simulink model "sampleModel1488"  (R2023a)
settings: Solver=VariableStepAuto  StartTime=0.0  StopTime=10.0  RelTol=1e-3
undefined symbols (not defined in the file): b011101a, b0c8, bf87616c, DiscIntNeverNeededParam, Newton, Raphson
libraries: simulink x171, slpidlib x32, simulink_need_slupdate x2
(part 2 of 6)

== system sampleModel1488/cfblk140 ==
  cfblk1 : Inport
  cfblk9 : Inport  Port=2
  cfblk10 : Inport  Port=3
  cfblk11 : Inport  Port=4
  cfblk14 : Delay  SampleTime=1
  cfblk3 : simulink/Discrete/Tapped Delay  vinit=0.0  samptime=-1  NumDelays=1  DelayOrder=Oldest  includeCurrent=off
  cfblk4 : Delay  SampleTime=1
  cfblk5 : Assignment  DiagnosticForDimensions=Warning  IndexOptions=Index vector (dialog)  Indices=1  OutputSizes=1
  cfblk6 : Gain  Gain=[-337675472.519738]
  cfblk7 : Subsystem
  cfblk8 : Subsystem
  cfblk2 : Outport
  cfblk12 : Outport  Port=2
  cfblk13 : Outport  Port=3
  wires:
  cfblk1/1 -> cfblk12/1
  cfblk8/1(cfblk2) -> cfblk2/1
  cfblk4/1 -> cfblk6/1
  cfblk9/1 -> cfblk4/1
  cfblk10/1 -> cfblk7/1(cfblk1)
  cfblk3/1 -> cfblk8/1(cfblk1)
  cfblk11/1 -> cfblk5/1
  cfblk8/2(cfblk11) -> cfblk5/2
  cfblk6/1 -> cfblk7/2(cfblk11), cfblk7/3(cfblk12)
  cfblk7/1(cfblk2) -> cfblk8/2(cfblk10)
  cfblk7/2(cfblk13) -> cfblk13/1
  cfblk5/1 -> cfblk14/1
  cfblk14/1 -> cfblk3/1

== system sampleModel1488/cfblk141 ==
  cfblk1 : Inport
  cfblk12 : Inport  Port=2
  cfblk13 : Inport  Port=3
  cfblk10 : Subsystem
  cfblk11 : Subsystem
  cfblk14 : Delay  SampleTime=1
  cfblk15 : Delay  SampleTime=1
  cfblk3 : Delay  SampleTime=1
  cfblk4 : PermuteDimensions
  cfblk5 : Signum
  cfblk6 : Math
  cfblk7 : Constant  Value=[773437629.546619]  SampleTime=1
  cfblk8 : Constant  Value=[-615309156.626634]  SampleTime=1
  cfblk9 : Subsystem
  cfblk2 : Outport
  wires:
  cfblk12/1 -> cfblk4/1
  cfblk11/2(cfblk7) -> cfblk10/1(cfblk1)
  cfblk8/1 -> cfblk2/1
  cfblk7/1 -> cfblk5/1
  cfblk1/1 -> cfblk9/2(cfblk7)
  cfblk13/1 -> cfblk9/3(cfblk8)
  cfblk9/1(cfblk2) -> cfblk3/1
  cfblk9/2(cfblk10) -> cfblk6/1
  cfblk4/1 -> cfblk11/1(cfblk1)
  cfblk9/3(cfblk11) -> cfblk11/2(cfblk6)
  cfblk11/1(cfblk2) -> cfblk14/1
  cfblk14/1 -> cfblk9/1(cfblk1)
  cfblk10/1(cfblk2) -> cfblk15/1
  cfblk15/1 -> cfblk9/4(cfblk9)

== system sampleModel1488/cfblk142 ==
  cfblk1 : Inport
  cfblk8 : Inport  Port=2
  cfblk{10..14} (5 alike) : Delay  SampleTime=1
  cfblk3 : Constant  Value=[-728485137.526243]  SampleTime=1
  cfblk4 : Subsystem
  cfblk5 : Subsystem
  cfblk6 : Subsystem
  cfblk7 : Subsystem
  cfblk2 : Outport
  cfblk9 : Outport  Port=2
  wires:
  cfblk8/1 -> cfblk2/1, cfblk6/3(cfblk13), cfblk6/6(cfblk16)
  cfblk5/1(cfblk2) -> cfblk7/1(cfblk1)
  cfblk1/1 -> cfblk4/1(cfblk1), cfblk6/2(cfblk12)
  cfblk5/2(cfblk8) -> cfblk13/1, cfblk14/1
  cfblk3/1 -> cfblk4/3(cfblk14)
  cfblk4/1(cfblk2) -> cfblk9/1
  cfblk6/1(cfblk2) -> cfblk5/2(cfblk6)
  cfblk4/2(cfblk15) -> cfblk6/1(cfblk1)
  cfblk7/2(cfblk15) -> cfblk11/1, cfblk12/1
  cfblk7/1(cfblk2) -> cfblk10/1
  cfblk10/1 -> cfblk5/1(cfblk1)
  cfblk11/1 -> cfblk5/3(cfblk7)
  cfblk12/1 -> cfblk6/5(cfblk15)
  cfblk13/1 -> cfblk4/2(cfblk13)
  cfblk14/1 -> cfblk6/4(cfblk14)

== system sampleModel1488/cfblk143 ==
  cfblk1 : Inport
  cfblk11 : Inport  Port=2
  cfblk10 : Subsystem
  cfblk12 : Delay  SampleTime=1
  cfblk13 : Delay  SampleTime=1
  cfblk3 : simulink/Discrete/Transfer Fcn First Order  PoleZ=0.95  ICPrevOutput=0.0  DoSatur=off
  cfblk4 : DiscreteFir  SampleTime=1
  cfblk5 : Squeeze
  cfblk6 : ComplexToRealImag
  cfblk7 : Subsystem
  cfblk8 : Subsystem
  cfblk9 : Subsystem
  cfblk2 : Outport
  wires:
  cfblk1/1 -> cfblk9/1(cfblk1)
  cfblk8/1(cfblk2) -> cfblk6/1
  cfblk8/2(cfblk8) -> cfblk2/1
  cfblk4/1 -> cfblk10/1(cfblk1)
  cfblk9/1(cfblk2) -> cfblk4/1
  cfblk7/1(cfblk2) -> cfblk5/1
  cfblk10/1(cfblk2) -> cfblk3/1
  cfblk5/1 -> cfblk8/1(cfblk1)
  cfblk7/2(cfblk13) -> cfblk8/2(cfblk7)
  cfblk11/1 -> cfblk7/1(cfblk1)
  cfblk9/2(cfblk12) -> cfblk7/2(cfblk9)
  cfblk3/1 -> cfblk7/3(cfblk10)
  cfblk10/2(cfblk8) -> cfblk7/5(cfblk12)
  cfblk6/1 -> cfblk12/1
  cfblk12/1 -> cfblk10/2(cfblk7)
  cfblk6/2 -> cfblk13/1
  cfblk13/1 -> cfblk7/4(cfblk11)

== system sampleModel1488/cfblk144 ==
  cfblk1 : Inport
  cfblk3 : DiscreteZeroPole  Poles=[0 0.5]  Gain=1
  cfblk4 : DiscreteZeroPole  Poles=[0 0.5]  Gain=1
  cfblk5 : Polyval  Coefs=[ +2.081618890e-019, -1.441693666e-014, +4.719686976e-010, -8.536869453e-006, +1.621573104e-001, -8.087801117e+001 ]
  cfblk6 : Signum
  cfblk7 : Product  Inputs=**
  cfblk9 : Delay  SampleTime=1
  cfblk2 : Outport
  cfblk8 : Outport  Port=2
  wires:
  cfblk5/1 -> cfblk2/1
  cfblk4/1 -> cfblk6/1
  cfblk7/1 -> cfblk4/1
  cfblk3/1 -> cfblk8/1, cfblk9/1
  cfblk6/1 -> cfblk3/1, cfblk5/1
  cfblk1/1 -> cfblk7/2
  cfblk9/1 -> cfblk7/1

== system sampleModel1488/cfblk145 ==
  cfblk1 : Inport
  cfblk9 : Inport  Port=2
  cfblk10 : Inport  Port=3
  cfblk11 : Inport  Port=4
  cfblk12 : Delay  SampleTime=1
  cfblk13 : Delay  SampleTime=1
  cfblk3 : Delay  DelayLengthSource=Input port  SampleTime=1
      settings: InputPortMap=u0,p1
  cfblk4 : DiscreteFilter  SampleTime=1
  cfblk5 : Bias  Bias=[63106106.274420]  SaturateOnIntegerOverflow=off
  cfblk6 : Constant  Value=[428304277.338585]  SampleTime=1
  cfblk7 : Subsystem
  cfblk8 : Subsystem
  cfblk2 : Outport
  wires:
  cfblk11/1 -> cfblk3/1
  cfblk6/1 -> cfblk7/1(cfblk1)
  cfblk5/1 -> cfblk7/2(cfblk11)
  cfblk9/1 -> cfblk2/1
  cfblk4/1 -> cfblk8/1(cfblk1)
  cfblk10/1 -> cfblk8/2(cfblk9)
  cfblk8/1(cfblk2) -> cfblk5/1
  cfblk1/1 -> cfblk3/2
  cfblk7/1(cfblk2) -> cfblk12/1
  cfblk12/1 -> cfblk4/1
  cfblk7/2(cfblk12) -> cfblk13/1
  cfblk13/1 -> cfblk8/3(cfblk10)

== system sampleModel1488/cfblk146 ==
  cfblk1 : Inport
  cfblk10 : Subsystem
  cfblk11 : Delay  SampleTime=1
  cfblk12 : Delay  SampleTime=1
  cfblk13 : Delay  SampleTime=1
  cfblk3 : simulink/Discrete/Transfer Fcn Real Zero  ZeroZ=0.75  ICPrevInput=0.0  DoSatur=off
  cfblk4 : Sqrt  Operator=rSqrt  AlgorithmType=Newton-Raphson
  cfblk5 : Constant  Value=[-692942058.607273]  SampleTime=1
  cfblk6 : Subsystem
  cfblk7 : Subsystem
  cfblk8 : Subsystem
  cfblk9 : Subsystem
  cfblk2 : Outport
  wires:
  cfblk10/1(cfblk2) -> cfblk6/2(cfblk12)
  cfblk8/1(cfblk2) -> cfblk3/1
  cfblk8/2(cfblk10) -> cfblk9/1(cfblk1)
  cfblk1/1 -> cfblk7/2(cfblk9)
  cfblk6/1(cfblk2) -> cfblk4/1
  cfblk7/1(cfblk2) -> cfblk2/1
  cfblk7/2(cfblk10) -> cfblk8/1(cfblk1)
  cfblk9/3(cfblk15) -> cfblk10/1(cfblk1)
  cfblk3/1 -> cfblk10/2(cfblk9)
  cfblk4/1 -> cfblk11/1
  cfblk11/1 -> cfblk6/1(cfblk1)
  cfblk9/1(cfblk2) -> cfblk12/1
  cfblk12/1 -> cfblk7/1(cfblk1)
  cfblk9/2(cfblk14) -> cfblk13/1
  cfblk13/1 -> cfblk8/2(cfblk9)

== system sampleModel1488/cfblk147 ==
  cfblk1 : Inport
  cfblk10 : Subsystem
  cfblk11 : Subsystem
  cfblk{12..15} (4 alike) : Delay  SampleTime=1
  cfblk3 : Delay  ShowEnablePort=on  SampleTime=1
      settings: InputPortMap=u0,e6
  cfblk4 : UnitDelay  HasFrameUpgradeWarning=on
  cfblk5 : Sum  Inputs=+
  cfblk6 : Assignment  DiagnosticForDimensions=Warning  IndexOptions=Index vector (dialog)  Indices=1  OutputSizes=1
  cfblk7 : PermuteDimensions
  cfblk8 : Constant  Value=[-634312519.623233]  SampleTime=1
  cfblk9 : Subsystem
  cfblk2 : Outport
  wires:
  cfblk3/1 -> cfblk5/1
  cfblk4/1 -> cfblk10/1(cfblk1), cfblk9/3(cfblk8)
  cfblk11/1(cfblk2) -> cfblk3/1
  cfblk11/2(cfblk8) -> cfblk7/1
  cfblk1/1 -> cfblk2/1, cfblk11/3(cfblk6), cfblk11/4(cfblk7)
  cfblk9/1(cfblk2) -> cfblk13/1, cfblk14/1
  cfblk10/1(cfblk2) -> cfblk9/5(cfblk10), cfblk12/1
  cfblk7/1 -> cfblk4/1
  cfblk5/1 -> cfblk10/3(cfblk9)
  cfblk8/1 -> cfblk6/1, cfblk9/1(cfblk1), cfblk9/2(cfblk7), cfblk10/4(cfblk10)
  cfblk11/3(cfblk9) -> cfblk6/2, cfblk9/4(cfblk9)
  cfblk12/1 -> cfblk3/2
  cfblk13/1 -> cfblk10/2(cfblk8)
  cfblk14/1 -> cfblk11/2(cfblk5)
  cfblk6/1 -> cfblk15/1
  cfblk15/1 -> cfblk11/1(cfblk1)

== system sampleModel1488/cfblk148 ==
  cfblk1 : Inport
  cfblk{10..17} (8 alike) : Delay  SampleTime=1
  cfblk3 : simulink/Math Operations/MinMax Running Resettable  Function=min  vinit=0.0
  cfblk4 : PermuteDimensions
  cfblk5 : Polyval  Coefs=[ +2.081618890e-019, -1.441693666e-014, +4.719686976e-010, -8.536869453e-006, +1.621573104e-001, -8.087801117e+001 ]
  cfblk6 : ComplexToRealImag
  cfblk7 : Subsystem
  cfblk8 : Subsystem
  cfblk2 : Outport
  cfblk9 : Outport  Port=2
  wires:
  cfblk7/1(cfblk2) -> cfblk8/1(cfblk1)
  cfblk1/1 -> cfblk7/1(cfblk1)
  cfblk3/1 -> cfblk4/1, cfblk14/1
  cfblk5/1 -> cfblk3/1, cfblk15/1
  cfblk8/1(cfblk2) -> cfblk2/1
  cfblk7/2(cfblk14) -> cfblk6/1
  cfblk4/1 -> cfblk10/1, cfblk11/1, cfblk12/1, cfblk13/1
  cfblk6/1 -> cfblk9/1
  cfblk8/2(cfblk13) -> cfblk5/1, cfblk16/1
  cfblk10/1 -> cfblk8/2(cfblk10)
  cfblk11/1 -> cfblk3/2
  cfblk12/1 -> cfblk8/3(cfblk11)
  cfblk13/1 -> cfblk7/4(cfblk12)
  cfblk14/1 -> cfblk8/4(cfblk12)
  cfblk15/1 -> cfblk7/3(cfblk11)
  cfblk16/1 -> cfblk7/5(cfblk13)
  cfblk6/2 -> cfblk17/1
  cfblk17/1 -> cfblk7/2(cfblk10)

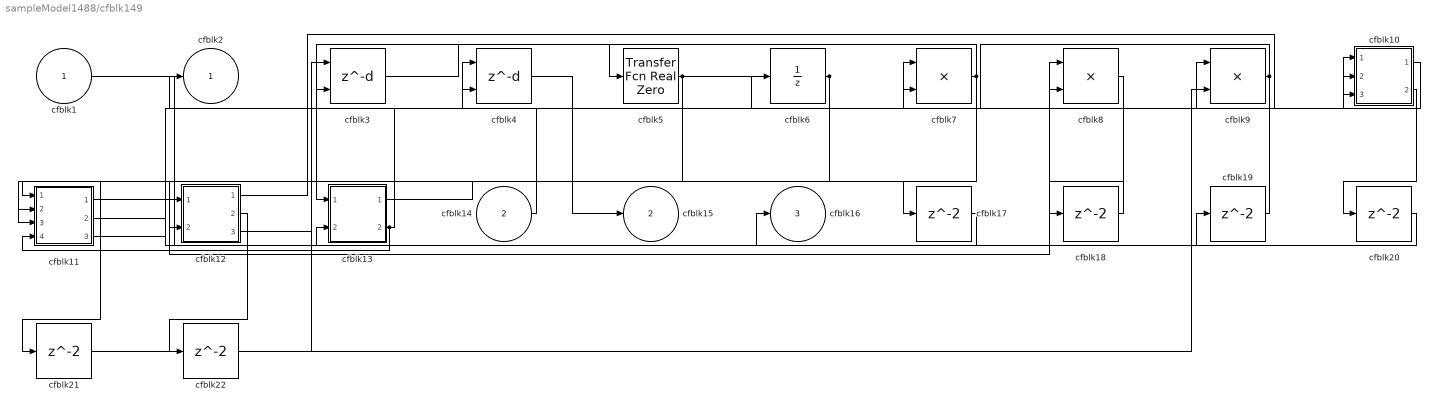
== system sampleModel1488/cfblk149 ==
  cfblk1 : Inport
  cfblk14 : Inport  Port=2
  cfblk10 : Subsystem
  cfblk11 : Subsystem
  cfblk12 : Subsystem
  cfblk13 : Subsystem
  cfblk{17..22} (6 alike) : Delay  SampleTime=1
  cfblk3 : Delay  DelayLengthSource=Input port  SampleTime=1
      settings: InputPortMap=u0,p1
  cfblk4 : Delay  DelayLengthSource=Input port  SampleTime=1
      settings: InputPortMap=u0,p1
  cfblk5 : simulink/Discrete/Transfer Fcn Real Zero  ZeroZ=0.75  ICPrevInput=0.0  DoSatur=off
  cfblk6 : UnitDelay  HasFrameUpgradeWarning=on
  cfblk7 : Product
  cfblk8 : Product
  cfblk9 : Product  Inputs=**
  cfblk2 : Outport
  cfblk15 : Outport  Port=2
  cfblk16 : Outport  Port=3
  wires:
  cfblk14/1 -> cfblk4/1
  cfblk7/1 -> cfblk13/1(cfblk1), cfblk11/3(cfblk14), cfblk21/1
  cfblk1/1 -> cfblk16/1
  cfblk11/1(cfblk2) -> cfblk8/1
  cfblk9/1 -> cfblk7/1, cfblk8/2
  cfblk4/1 -> cfblk15/1
  cfblk12/1(cfblk2) -> cfblk9/1
  cfblk6/1 -> cfblk12/1(cfblk1), cfblk11/1(cfblk1)
  cfblk12/3(cfblk10) -> cfblk10/1(cfblk1)
  cfblk10/1(cfblk2) -> cfblk4/2
  cfblk5/1 -> cfblk6/1, cfblk11/2(cfblk13), cfblk10/3(cfblk10)
  cfblk3/1 -> cfblk5/1
  cfblk11/3(cfblk17) -> cfblk10/2(cfblk9)
  cfblk13/2(cfblk15) -> cfblk2/1, cfblk11/4(cfblk15)
  cfblk13/1(cfblk2) -> cfblk17/1
  cfblk17/1 -> cfblk12/2(cfblk8)
  cfblk8/1 -> cfblk18/1
  cfblk18/1 -> cfblk7/2
  cfblk11/2(cfblk16) -> cfblk19/1
  cfblk19/1 -> cfblk3/2
  cfblk10/2(cfblk11) -> cfblk20/1
  cfblk20/1 -> cfblk13/2(cfblk14)
  cfblk21/1 -> cfblk9/2
  cfblk12/2(cfblk9) -> cfblk22/1
  cfblk22/1 -> cfblk3/1

== system sampleModel1488/cfblk150 ==
  cfblk1 : Inport
  cfblk10 : Inport  Port=2
  cfblk11 : Inport  Port=3
  cfblk12 : Inport  Port=4
  cfblk14 : Delay  SampleTime=1
  cfblk15 : Delay  SampleTime=1
  cfblk16 : Delay  SampleTime=1
  cfblk3 : Delay  DelayLengthSource=Input port  SampleTime=1
      settings: InputPortMap=u0,p1
  cfblk4 : Delay  ShowEnablePort=on  SampleTime=1
      settings: InputPortMap=u0,e6
  cfblk5 : Delay  ShowEnablePort=on  SampleTime=1
      settings: InputPortMap=u0,e6
  cfblk6 : Product
  cfblk7 : Sum  Inputs=--
  cfblk8 : Subsystem
  cfblk9 : Subsystem
  cfblk2 : Outport
  cfblk13 : Outport  Port=2
  wires:
  cfblk9/1(cfblk2) -> cfblk3/1
  cfblk8/1(cfblk2) -> cfblk9/1(cfblk1)
  cfblk3/1 -> cfblk5/1, cfblk4/2, cfblk15/1
  cfblk9/2(cfblk15) -> cfblk6/1
  cfblk12/1 -> cfblk13/1, cfblk8/4(cfblk15), cfblk8/5(cfblk16)
  cfblk11/1 -> cfblk5/2
  cfblk4/1 -> cfblk7/1
  cfblk7/1 -> cfblk2/1
  cfblk1/1 -> cfblk8/2(cfblk13), cfblk7/2, cfblk6/2
  cfblk9/3(cfblk16) -> cfblk3/2
  cfblk10/1 -> cfblk4/1
  cfblk5/1 -> cfblk14/1
  cfblk14/1 -> cfblk8/1(cfblk1)
  cfblk15/1 -> cfblk8/3(cfblk14)
  cfblk6/1 -> cfblk16/1
  cfblk16/1 -> cfblk9/2(cfblk14)

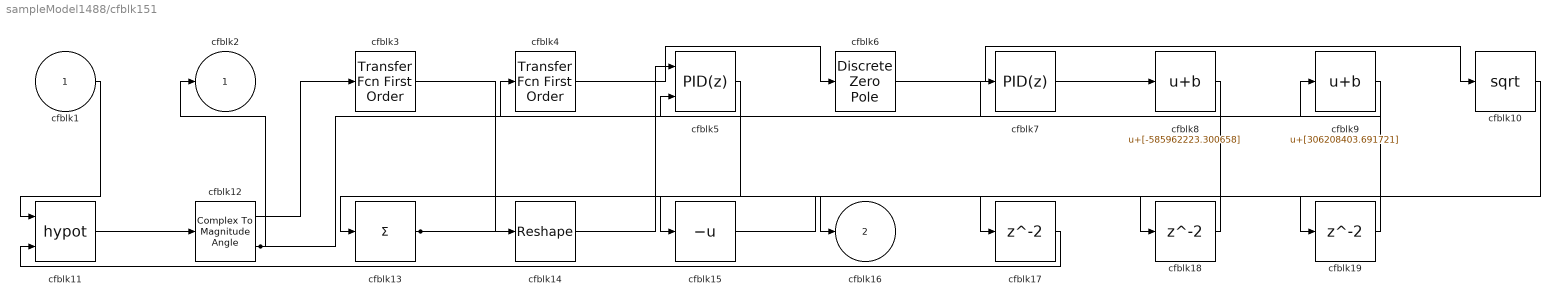
== system sampleModel1488/cfblk151 ==
  cfblk1 : Inport
  cfblk10 : Sqrt
  cfblk11 : Math  Operator=hypot
  cfblk12 : ComplexToMagnitudeAngle
  cfblk13 : Sum  Inputs=+
  cfblk14 : Reshape
  cfblk15 : UnaryMinus
  cfblk17 : Delay  SampleTime=1
  cfblk18 : Delay  SampleTime=1
  cfblk19 : Delay  SampleTime=1
  cfblk3 : simulink/Discrete/Transfer Fcn First Order  PoleZ=0.95  ICPrevOutput=0.0  DoSatur=off
  cfblk4 : simulink/Discrete/Transfer Fcn First Order  PoleZ=0.95  ICPrevOutput=0.0  DoSatur=off
  cfblk5 : slpidlib/PID Controller (2DOF)  Controller=PID  Form=Parallel  TimeDomain=Discrete-time  UseExternalTs=off  SampleTime=1  IntegratorMethod=Forward Euler  FilterMethod=Forward Euler  ControllerParametersSource=internal  P=1  I=1  UseKiTs=off  D=0  N=100  UseFilter=on  b=1  c=1  TunerSelectOption=Transfer Function Based (PID Tuner App)  InitialConditionSource=internal  InitialConditionForIntegrator=0  InitialConditionForFilter=0  DifferentiatorICPrevScaledInput=0  ExternalReset=none  TrackingMode=off  Kt=1  LimitOutput=off  SatLimitsSource=internal  UpperSaturationLimit=inf  LowerSaturationLimit=-inf  LinearizeAsGain=off  AntiWindupMode=none  Kb=1  LimitIntegrator=off  UpperIntegratorSaturationLimit=inf  LowerIntegratorSaturationLimit=-inf  POutMin=[]  POutMax=[]  IOutMin=[]  IOutMax=[]  DOutMin=[]  DOutMax=[]  NOutMin=[]  NOutMax=[]  bOutMin=[]  bOutMax=[]  cOutMin=[]  cOutMax=[]  SumOutMin=[]  SumOutMax=[]  SaturationOutMin=[]  SaturationOutMax=[]  PParamMin=[]  PParamMax=[]  IParamMin=[]  IParamMax=[]  DParamMin=[]  DParamMax=[]  NParamMin=[]  NParamMax=[]  bParamMin=[]  bParamMax=[]  cParamMin=[]  cParamMax=[]  KbParamMin=[]  KbParamMax=[]  KtParamMin=[]  KtParamMax=[]  KbOutMin=[]  KbOutMax=[]  KtOutMin=[]  KtOutMax=[]  IntegratorOutMin=[]  IntegratorOutMax=[]  FilterOutMin=[]  FilterOutMax=[]  SumI1OutMin=[]  SumI1OutMax=[]  SumI2OutMin=[]  SumI2OutMax=[]  SumI3OutMin=[]  SumI3OutMax=[]  SumI4OutMin=[]  SumI4OutMax=[]  SumDOutMin=[]  SumDOutMax=[]  Sum1OutMin=[]  Sum1OutMax=[]  Sum2OutMin=[]  Sum2OutMax=[]  Sum3OutMin=[]  Sum3OutMax=[]  DifferentiatorOutMin=[]  DifferentiatorOutMax=[]  FilterDiffOutCoefMin=[]  FilterDiffOutCoefMax=[]  ReciprocalOutMin=[]  ReciprocalOutMax=[]  SumDenOutMin=[]  SumDenOutMax=[]  SumNumOutMin=[]  SumNumOutMax=[]  DivideOutMin=[]  DivideOutMax=[]  UdiffTsProdOutMin=[]  UdiffTsProdOutMax=[]  NTsProdOutMin=[]  NTsProdOutMax=[]  UintegralTsProdOutMin=[]  UintegralTsProdOutMax=[]  UngainTsProdOutMin=[]  UngainTsProdOutMax=[]  ClampingZeroOutDataTypeStr=Inherit: Inherit via back propagation  ClampingZeroOutMin=[]  ClampingZeroOutMax=[]  FilterDenConstantOutDataTypeStr=Inherit: Inherit via back propagation  FilterDenConstantOutMin=[]  FilterDenConstantOutMax=[]  PCopyOutDataTypeStr=Inherit: Inherit via back propagation  PCopyOutMin=[]  PCopyOutMax=[]  NCopyOutDataTypeStr=Inherit: Inherit via back propagation  NCopyOutMin=[]  NCopyOutMax=[]  IntegratorContinuousStateAttributes=''  IntegratorStateMustResolveToSignalObject=off  IntegratorRTWStateStorageClass=Auto  FilterContinuousStateAttributes=''  FilterStateMustResolveToSignalObject=off  FilterRTWStateStorageClass=Auto  ParallelPVariant=InternalParameters  IdealPVariant=Disabled  IVariant=InternalParameters  DVariant=InternalParameters  bVariant=InternalParameters  cVariant=InternalParameters  IntegratorVariant=Discrete  SatVariant=Disabled  AWVariant=Passthrough  PCopyVariant=Disabled  TRVariant=Disabled  FdbkBlocksVariant=Forward  IdealPFdbkVariant=Disabled  SatFdbkVariant=Disabled  DerivativeFilterVariant=ForwardEulerFilter  NVariant=InternalParameters  NCopyVariant=Disabled  FilterICVariant=InternalICsFilter  IntegratorICVariant=InternalICs  ExternalResetVariant=Disabled  TRSumVariant=Passthrough  SumFdbkVariant=Disabled  SumVariant=Sum_PID  TsampFilterVariant=InternalTs  TsampNgainVariant=Passthrough  TsampIntegralVariant=Disabled_SignalSpec  ExternalSaturationOutDataTypeStr=Inherit: Same as second input
      settings: LibrarySourceBlock=simulink/Discrete/Discrete PID Controller (2DOF)
  cfblk6 : DiscreteZeroPole  Poles=[0 0.5]  Gain=1
  cfblk7 : slpidlib/PID Controller  Controller=PID  Form=Parallel  TimeDomain=Discrete-time  UseExternalTs=off  SampleTime=1  IntegratorMethod=Forward Euler  FilterMethod=Forward Euler  ControllerParametersSource=internal  P=1  I=1  UseKiTs=off  D=0  N=100  UseFilter=on  TunerSelectOption=Transfer Function Based (PID Tuner App)  InitialConditionSource=internal  InitialConditionForIntegrator=0  InitialConditionForFilter=0  DifferentiatorICPrevScaledInput=0  ExternalReset=none  TrackingMode=off  Kt=1  LimitOutput=off  SatLimitsSource=internal  UpperSaturationLimit=inf  LowerSaturationLimit=-inf  LinearizeAsGain=off  AntiWindupMode=none  Kb=1  LimitIntegrator=off  UpperIntegratorSaturationLimit=inf  LowerIntegratorSaturationLimit=-inf  POutMin=[]  POutMax=[]  IOutMin=[]  IOutMax=[]  DOutMin=[]  DOutMax=[]  NOutMin=[]  NOutMax=[]  SumOutMin=[]  SumOutMax=[]  SaturationOutMin=[]  SaturationOutMax=[]  PParamMin=[]  PParamMax=[]  IParamMin=[]  IParamMax=[]  DParamMin=[]  DParamMax=[]  NParamMin=[]  NParamMax=[]  KbParamMin=[]  KbParamMax=[]  KtParamMin=[]  KtParamMax=[]  KbOutMin=[]  KbOutMax=[]  KtOutMin=[]  KtOutMax=[]  IntegratorOutMin=[]  IntegratorOutMax=[]  FilterOutMin=[]  FilterOutMax=[]  SumI1OutMin=[]  SumI1OutMax=[]  SumI2OutMin=[]  SumI2OutMax=[]  SumI3OutMin=[]  SumI3OutMax=[]  SumI4OutMin=[]  SumI4OutMax=[]  SumDOutMin=[]  SumDOutMax=[]  DifferentiatorOutMin=[]  DifferentiatorOutMax=[]  FilterDiffOutCoefMin=[]  FilterDiffOutCoefMax=[]  ReciprocalOutMin=[]  ReciprocalOutMax=[]  SumDenOutMin=[]  SumDenOutMax=[]  SumNumOutMin=[]  SumNumOutMax=[]  DivideOutMin=[]  DivideOutMax=[]  UdiffTsProdOutMin=[]  UdiffTsProdOutMax=[]  NTsProdOutMin=[]  NTsProdOutMax=[]  UintegralTsProdOutMin=[]  UintegralTsProdOutMax=[]  UngainTsProdOutMin=[]  UngainTsProdOutMax=[]  ClampingZeroOutDataTypeStr=Inherit: Inherit via back propagation  ClampingZeroOutMin=[]  ClampingZeroOutMax=[]  FilterDenConstantOutDataTypeStr=Inherit: Inherit via back propagation  FilterDenConstantOutMin=[]  FilterDenConstantOutMax=[]  PCopyOutDataTypeStr=Inherit: Inherit via back propagation  PCopyOutMin=[]  PCopyOutMax=[]  NCopyOutDataTypeStr=Inherit: Inherit via back propagation  NCopyOutMin=[]  NCopyOutMax=[]  IntegratorContinuousStateAttributes=''  IntegratorStateMustResolveToSignalObject=off  IntegratorRTWStateStorageClass=Auto  FilterContinuousStateAttributes=''  FilterStateMustResolveToSignalObject=off  FilterRTWStateStorageClass=Auto  ParallelPVariant=InternalParameters  IdealPVariant=Disabled  IVariant=InternalParameters  DVariant=InternalParameters  IntegratorVariant=Discrete  SatVariant=Disabled  AWVariant=Passthrough  PCopyVariant=Disabled  TRVariant=Disabled  FdbkBlocksVariant=Forward  IdealPFdbkVariant=Disabled  SatFdbkVariant=Disabled  DerivativeFilterVariant=ForwardEulerFilter  NVariant=InternalParameters  NCopyVariant=Disabled  FilterICVariant=InternalICsFilter  IntegratorICVariant=InternalICs  ExternalResetVariant=Disabled  TRSumVariant=Passthrough  SumFdbkVariant=Disabled  SumVariant=Sum_PID  TsampFilterVariant=InternalTs  TsampNgainVariant=Passthrough  TsampIntegralVariant=Disabled_SignalSpec  ExternalSaturationOutDataTypeStr=Inherit: Same as second input
      settings: LibrarySourceBlock=simulink/Discrete/Discrete PID Controller
  cfblk8 : Bias  Bias=[-585962223.300658]  SaturateOnIntegerOverflow=off
  cfblk9 : Bias  Bias=[306208403.691721]  SaturateOnIntegerOverflow=off
  cfblk2 : Outport
  cfblk16 : Outport  Port=2
  wires:
  cfblk6/1 -> cfblk10/1
  cfblk9/1 -> cfblk4/1
  cfblk4/1 -> cfblk6/1
  cfblk7/1 -> cfblk8/1
  cfblk11/1 -> cfblk12/1
  cfblk5/1 -> cfblk15/1
  cfblk12/1 -> cfblk3/1
  cfblk12/2 -> cfblk2/1, cfblk5/2
  cfblk1/1 -> cfblk11/1
  cfblk13/1 -> cfblk14/1, cfblk19/1
  cfblk10/1 -> cfblk16/1
  cfblk14/1 -> cfblk9/1
  cfblk8/1 -> cfblk13/1
  cfblk3/1 -> cfblk17/1
  cfblk17/1 -> cfblk11/2
  cfblk15/1 -> cfblk18/1
  cfblk18/1 -> cfblk5/1
  cfblk19/1 -> cfblk7/1

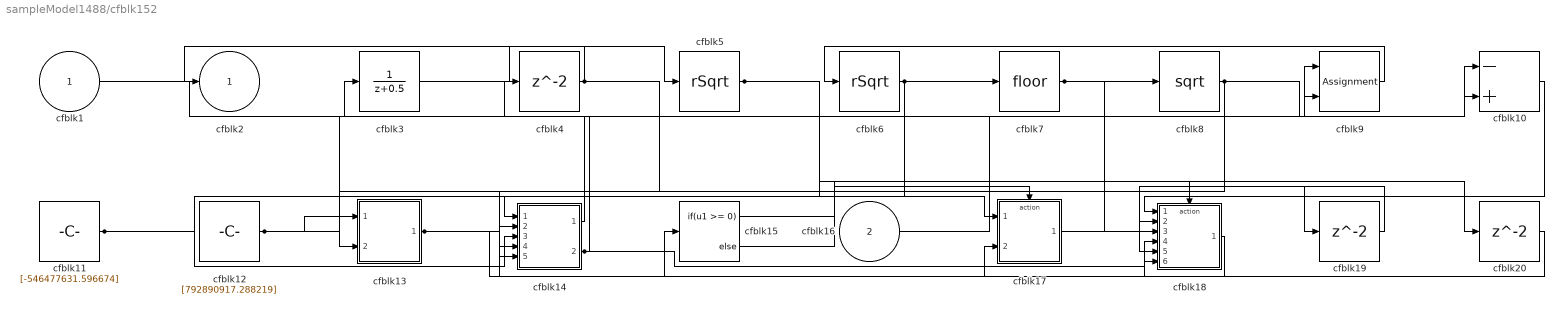
== system sampleModel1488/cfblk152 ==
  cfblk1 : Inport
  cfblk16 : Inport  Port=2
  cfblk10 : Sum  Inputs=-+
  cfblk11 : Constant  Value=[-546477631.596674]  SampleTime=1
  cfblk12 : Constant  Value=[792890917.288219]  SampleTime=1
  cfblk13 : Subsystem
  cfblk14 : Subsystem
  cfblk15 : If  IfExpression=u1 >= 0  SampleTime=1
  cfblk17 : Subsystem  TreatAsAtomicUnit=on
  cfblk18 : Subsystem  TreatAsAtomicUnit=on
  cfblk19 : Delay  SampleTime=1
  cfblk20 : Delay  SampleTime=1
  cfblk3 : DiscreteTransferFcn  SampleTime=1
  cfblk4 : Delay  SampleTime=1
  cfblk5 : Sqrt  Operator=rSqrt  AlgorithmType=Newton-Raphson
  cfblk6 : Sqrt  Operator=rSqrt  AlgorithmType=Newton-Raphson
  cfblk7 : Rounding
  cfblk8 : Sqrt
  cfblk9 : Assignment  DiagnosticForDimensions=Warning  IndexOptions=Index vector (dialog)  Indices=1  OutputSizes=1
  cfblk2 : Outport
  wires:
  cfblk7/1 -> cfblk8/1, cfblk18/3(cfblk14)
  cfblk3/1 -> cfblk5/1
  cfblk10/1 -> cfblk18/1(cfblk1)
  cfblk12/1 -> cfblk13/1(cfblk1), cfblk10/1
  cfblk9/1 -> cfblk6/1
  cfblk16/1 -> cfblk9/1
  cfblk14/1(cfblk2) -> cfblk4/1
  cfblk1/1 -> cfblk9/2
  cfblk5/1 -> cfblk17/1(cfblk1), cfblk20/1
  cfblk6/1 -> cfblk7/1, cfblk14/5(cfblk14)
  cfblk4/1 -> cfblk2/1, cfblk18/5(cfblk16)
  cfblk18/1(cfblk2) -> cfblk17/2(cfblk17)
  cfblk11/1 -> cfblk14/1(cfblk1), cfblk14/3(cfblk12)
  cfblk8/1 -> cfblk14/2(cfblk11), cfblk13/2(cfblk11), cfblk10/2
  cfblk13/1(cfblk2) -> cfblk15/1, cfblk18/4(cfblk15)
  cfblk14/2(cfblk15) -> cfblk3/1, cfblk18/6(cfblk17)
  cfblk15/1 -> cfblk17/Action
  cfblk15/2 -> cfblk18/Action
  cfblk17/1(cfblk2) -> cfblk19/1
  cfblk19/1 -> cfblk18/2(cfblk13)
  cfblk20/1 -> cfblk14/4(cfblk13)

== system sampleModel1488/cfblk153 ==
  cfblk1 : Inport
  cfblk13 : Inport  Port=2
  cfblk14 : Inport  Port=3
  cfblk15 : Inport  Port=4
  cfblk10 : Subsystem
  cfblk11 : Subsystem
  cfblk12 : Subsystem
  cfblk18 : Delay  SampleTime=1
  cfblk3 : DiscreteZeroPole  Poles=[0 0.5]  Gain=1
  cfblk4 : MinMax  Function=max  Inputs=2
  cfblk5 : Abs  SaturateOnIntegerOverflow=off
  cfblk6 : ComplexToRealImag
  cfblk7 : Constant  Value=[463129782.283015]  SampleTime=1
  cfblk8 : Subsystem
  cfblk9 : Subsystem
  cfblk2 : Outport
  cfblk16 : Outport  Port=2
  cfblk17 : Outport  Port=3
  wires:
  cfblk5/1 -> cfblk12/1(cfblk1), cfblk10/4(cfblk10)
  cfblk15/1 -> cfblk4/1
  cfblk14/1 -> cfblk6/1
  cfblk3/1 -> cfblk16/1
  cfblk13/1 -> cfblk12/2(cfblk9)
  cfblk11/1(cfblk2) -> cfblk10/1(cfblk1)
  cfblk6/1 -> cfblk5/1
  cfblk7/1 -> cfblk11/1(cfblk1)
  cfblk4/1 -> cfblk11/2(cfblk12)
  cfblk12/1(cfblk2) -> cfblk10/2(cfblk8)
  cfblk6/2 -> cfblk17/1
  cfblk12/2(cfblk10) -> cfblk4/2
  cfblk10/1(cfblk2) -> cfblk3/1
  cfblk1/1 -> cfblk8/1(cfblk1)
  cfblk9/1(cfblk2) -> cfblk2/1
  cfblk8/1(cfblk2) -> cfblk9/1(cfblk1)
  cfblk8/2(cfblk10) -> cfblk9/2(cfblk7)
  cfblk9/2(cfblk8) -> cfblk10/3(cfblk9)
  cfblk10/2(cfblk11) -> cfblk18/1
  cfblk18/1 -> cfblk8/2(cfblk9)

== system sampleModel1488/cfblk154 ==
  cfblk1 : Inport
  cfblk11 : Delay  SampleTime=1
  cfblk3 : UnitDelay  HasFrameUpgradeWarning=on
  cfblk4 : Reshape
  cfblk5 : Gain  Gain=[-293251258.042605]
  cfblk6 : Constant  Value=[668066207.533989]  SampleTime=1
  cfblk7 : Subsystem
  cfblk2 : Outport
  cfblk8 : Outport  Port=2
  cfblk9 : Outport  Port=3
  cfblk10 : Outport  Port=4
  wires:
  cfblk7/1(cfblk2) -> cfblk2/1
  cfblk7/2(cfblk7) -> cfblk3/1, cfblk10/1
  cfblk6/1 -> cfblk5/1
  cfblk4/1 -> cfblk9/1
  cfblk5/1 -> cfblk4/1
  cfblk1/1 -> cfblk8/1, cfblk7/2(cfblk6)
  cfblk3/1 -> cfblk11/1
  cfblk11/1 -> cfblk7/1(cfblk1)

== system sampleModel1488/cfblk155 ==
  cfblk1 : Inport
  cfblk3 : Sin  TimeSource=Use external signal  SampleTime=0
  cfblk4 : Constant  Value=[215090549.744625]  SampleTime=1
  cfblk5 : Subsystem
  cfblk6 : Subsystem
  cfblk2 : Outport
  cfblk7 : Outport  Port=2
  cfblk8 : Outport  Port=3
  wires:
  cfblk4/1 -> cfblk6/1(cfblk1), cfblk7/1
  cfblk6/1(cfblk2) -> cfblk5/1(cfblk1)
  cfblk6/2(cfblk16) -> cfblk5/2(cfblk12)
  cfblk5/1(cfblk2) -> cfblk2/1
  cfblk3/1 -> cfblk8/1
  cfblk1/1 -> cfblk5/3(cfblk13), cfblk5/4(cfblk14)
  cfblk5/2(cfblk15) -> cfblk3/1

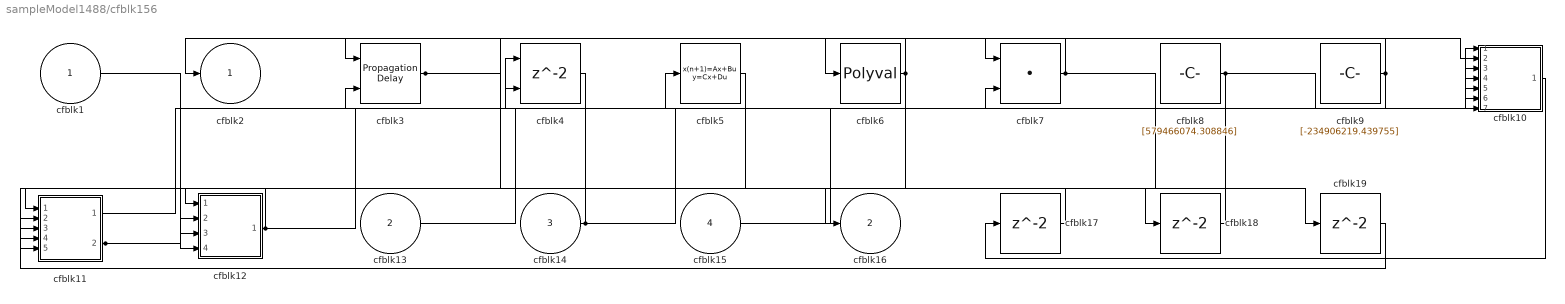
== system sampleModel1488/cfblk156 ==
  cfblk1 : Inport
  cfblk13 : Inport  Port=2
  cfblk14 : Inport  Port=3
  cfblk15 : Inport  Port=4
  cfblk10 : Subsystem
  cfblk11 : Subsystem
  cfblk12 : Subsystem
  cfblk17 : Delay  SampleTime=1
  cfblk18 : Delay  SampleTime=1
  cfblk19 : Delay  SampleTime=1
  cfblk3 : PropagationDelay  SampleTime=1
  cfblk4 : Delay  ShowEnablePort=on  SampleTime=1
      settings: InputPortMap=u0,e6
  cfblk5 : DiscreteStateSpace
  cfblk6 : Polyval  Coefs=[ +2.081618890e-019, -1.441693666e-014, +4.719686976e-010, -8.536869453e-006, +1.621573104e-001, -8.087801117e+001 ]
  cfblk7 : DotProduct  OutDataTypeStr=Inherit: Inherit via internal rule
  cfblk8 : Constant  Value=[579466074.308846]  SampleTime=1
  cfblk9 : Constant  Value=[-234906219.439755]  SampleTime=1
  cfblk2 : Outport
  cfblk16 : Outport  Port=2
  wires:
  cfblk7/1 -> cfblk2/1, cfblk6/1, cfblk19/1
  cfblk15/1 -> cfblk10/1(cfblk1)
  cfblk4/1 -> cfblk12/1(cfblk1)
  cfblk14/1 -> cfblk4/1, cfblk10/7(cfblk15)
  cfblk9/1 -> cfblk4/2, cfblk7/1
  cfblk5/1 -> cfblk12/3(cfblk10)
  cfblk6/1 -> cfblk3/1, cfblk16/1
  cfblk11/1(cfblk2) -> cfblk3/2
  cfblk3/1 -> cfblk10/2(cfblk10), cfblk18/1
  cfblk12/1(cfblk2) -> cfblk11/1(cfblk1), cfblk10/4(cfblk12)
  cfblk8/1 -> cfblk11/2(cfblk6), cfblk11/5(cfblk9), cfblk10/5(cfblk13)
  cfblk1/1 -> cfblk12/4(cfblk11)
  cfblk11/2(cfblk10) -> cfblk10/3(cfblk11), cfblk10/6(cfblk14), cfblk7/2
  cfblk13/1 -> cfblk5/1
  cfblk10/1(cfblk2) -> cfblk17/1
  cfblk17/1 -> cfblk12/2(cfblk9)
  cfblk18/1 -> cfblk11/3(cfblk7)
  cfblk19/1 -> cfblk11/4(cfblk8)

== system sampleModel1488/cfblk157 ==
  cfblk1 : Inport
  cfblk7 : Inport  Port=2
  cfblk8 : Inport  Port=3
  cfblk9 : Inport  Port=4
  cfblk10 : Inport  Port=5
  cfblk11 : Inport  Port=6
  cfblk12 : Subsystem  TreatAsAtomicUnit=on
  cfblk13 : Subsystem  TreatAsAtomicUnit=on
  cfblk{14..18} (5 alike) : Delay  SampleTime=1
  cfblk3 : DiscreteTransferFcn  SampleTime=1
  cfblk4 : DiscreteZeroPole  Poles=[0 0.5]  Gain=1
  cfblk5 : Product  Inputs=**
  cfblk6 : If  IfExpression=u1 >= 0  SampleTime=1
  cfblk2 : Outport
  wires:
  cfblk12/1(cfblk2) -> cfblk13/1(cfblk1)
  cfblk7/1 -> cfblk2/1
  cfblk1/1 -> cfblk6/1
  cfblk5/1 -> cfblk3/1
  cfblk3/1 -> cfblk4/1
  cfblk9/1 -> cfblk13/2(cfblk11)
  cfblk11/1 -> cfblk13/3(cfblk12)
  cfblk8/1 -> cfblk5/1
  cfblk10/1 -> cfblk13/4(cfblk13)
  cfblk13/3(cfblk15) -> cfblk5/2
  cfblk4/1 -> cfblk16/1, cfblk17/1
  cfblk6/1 -> cfblk12/Action
  cfblk6/2 -> cfblk13/Action
  cfblk13/1(cfblk2) -> cfblk14/1
  cfblk14/1 -> cfblk12/1(cfblk1)
  cfblk13/2(cfblk14) -> cfblk15/1
  cfblk15/1 -> cfblk12/2(cfblk5)
  cfblk16/1 -> cfblk12/3(cfblk6)
  cfblk17/1 -> cfblk12/5(cfblk8)
  cfblk13/4(cfblk16) -> cfblk18/1
  cfblk18/1 -> cfblk12/4(cfblk7)

== system sampleModel1488/cfblk158 ==
  cfblk1 : Inport
  cfblk13 : Inport  Port=2
  cfblk10 : Constant  Value=[-850657503.059018]  SampleTime=1
  cfblk11 : Subsystem
  cfblk12 : Subsystem
  cfblk15 : Delay  SampleTime=1
  cfblk3 : DiscreteFir  SampleTime=1
  cfblk4 : DiscreteFir  SampleTime=1
  cfblk5 : Reshape
  cfblk6 : simulink/Math Operations/MinMax Running Resettable  Function=min  vinit=0.0
  cfblk7 : Trigonometry
  cfblk8 : MinMax  Function=max
  cfblk9 : Constant  Value=[-933215899.881615]  SampleTime=1
  cfblk2 : Outport
  cfblk14 : Outport  Port=2
  wires:
  cfblk4/1 -> cfblk12/1(cfblk1), cfblk8/1
  cfblk7/1 -> cfblk5/1
  cfblk11/1(cfblk2) -> cfblk14/1
  cfblk10/1 -> cfblk6/1
  cfblk8/1 -> cfblk6/2
  cfblk6/1 -> cfblk3/1
  cfblk5/1 -> cfblk11/1(cfblk1)
  cfblk1/1 -> cfblk2/1
  cfblk13/1 -> cfblk11/2(cfblk15)
  cfblk3/1 -> cfblk7/1, cfblk11/4(cfblk17)
  cfblk9/1 -> cfblk11/3(cfblk16)
  cfblk12/1(cfblk2) -> cfblk15/1
  cfblk15/1 -> cfblk4/1

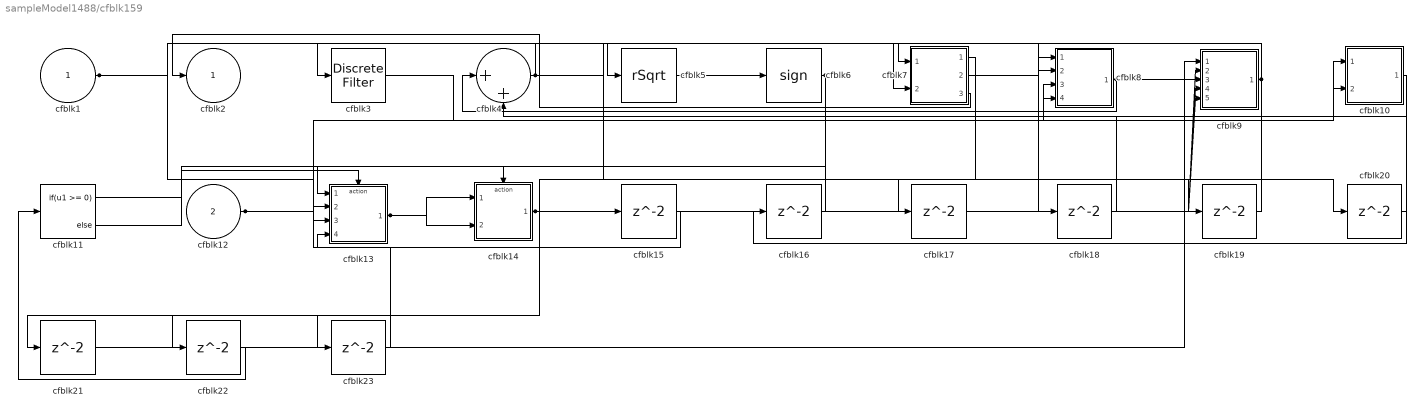
== system sampleModel1488/cfblk159 ==
  cfblk1 : Inport
  cfblk12 : Inport  Port=2
  cfblk10 : Subsystem
  cfblk11 : If  IfExpression=u1 >= 0  SampleTime=1
  cfblk13 : Subsystem  TreatAsAtomicUnit=on
  cfblk14 : Subsystem  TreatAsAtomicUnit=on
  cfblk{15..23} (9 alike) : Delay  SampleTime=1
  cfblk3 : DiscreteFilter  SampleTime=1
  cfblk4 : Sum  Inputs=|++
  cfblk5 : Sqrt  Operator=rSqrt  AlgorithmType=Newton-Raphson
  cfblk6 : Signum
  cfblk7 : Subsystem
  cfblk8 : Subsystem
  cfblk9 : Subsystem
  cfblk2 : Outport
  wires:
  cfblk4/1 -> cfblk3/1, cfblk7/1(cfblk1), cfblk19/1
  cfblk13/1(cfblk2) -> cfblk14/1(cfblk1), cfblk14/2(cfblk9)
  cfblk5/1 -> cfblk6/1
  cfblk8/1(cfblk2) -> cfblk4/1, cfblk20/1
  cfblk3/1 -> cfblk10/1(cfblk1)
  cfblk9/1(cfblk2) -> cfblk8/2(cfblk6), cfblk5/1, cfblk23/1
  cfblk14/1(cfblk2) -> cfblk9/2(cfblk7), cfblk9/4(cfblk9), cfblk9/5(cfblk10), cfblk15/1
  cfblk7/3(cfblk12) -> cfblk2/1
  cfblk1/1 -> cfblk13/3(cfblk14), cfblk7/2(cfblk10)
  cfblk6/1 -> cfblk21/1, cfblk22/1
  cfblk12/1 -> cfblk10/2(cfblk7), cfblk8/3(cfblk7)
  cfblk11/1 -> cfblk13/Action
  cfblk11/2 -> cfblk14/Action
  cfblk15/1 -> cfblk13/2(cfblk13)
  cfblk10/1(cfblk2) -> cfblk16/1
  cfblk16/1 -> cfblk13/1(cfblk1)
  cfblk7/1(cfblk2) -> cfblk17/1
  cfblk17/1 -> cfblk8/1(cfblk1)
  cfblk7/2(cfblk11) -> cfblk18/1
  cfblk18/1 -> cfblk4/2
  cfblk19/1 -> cfblk8/4(cfblk8)
  cfblk20/1 -> cfblk9/3(cfblk8)
  cfblk21/1 -> cfblk9/1(cfblk1)
  cfblk22/1 -> cfblk11/1
  cfblk23/1 -> cfblk13/4(cfblk15)

== system sampleModel1488/cfblk160 ==
  cfblk1 : Inport
  cfblk12 : Inport  Port=2
  cfblk13 : Inport  Port=3
  cfblk14 : Inport  Port=4
  cfblk10 : Subsystem
  cfblk11 : Subsystem
  cfblk{15..19} (5 alike) : Delay  SampleTime=1
  cfblk3 : Delay  ShowEnablePort=on  SampleTime=1
      settings: InputPortMap=u0,e6
  cfblk4 : Sum  Inputs=--
  cfblk5 : Math  Operator=transpose
  cfblk6 : Subsystem
  cfblk7 : Subsystem
  cfblk8 : Subsystem
  cfblk9 : Subsystem
  cfblk2 : Outport
  wires:
  cfblk12/1 -> cfblk9/1(cfblk1)
  cfblk10/1(cfblk2) -> cfblk5/1
  cfblk8/1(cfblk2) -> cfblk6/1(cfblk1)
  cfblk6/1(cfblk2) -> cfblk10/1(cfblk1)
  cfblk1/1 -> cfblk9/2(cfblk6)
  cfblk14/1 -> cfblk8/2(cfblk12)
  cfblk13/1 -> cfblk9/4(cfblk8)
  cfblk6/2(cfblk11) -> cfblk7/1(cfblk1)
  cfblk4/1 -> cfblk18/1, cfblk19/1
  cfblk3/1 -> cfblk10/2(cfblk8), cfblk7/3(cfblk14), cfblk16/1
  cfblk5/1 -> cfblk2/1
  cfblk8/3(cfblk16) -> cfblk11/1(cfblk1)
  cfblk9/1(cfblk2) -> cfblk8/4(cfblk14)
  cfblk6/3(cfblk12) -> cfblk3/1
  cfblk9/2(cfblk9) -> cfblk3/2
  cfblk8/4(cfblk17) -> cfblk6/2(cfblk8), cfblk7/2(cfblk13)
  cfblk11/1(cfblk2) -> cfblk4/1, cfblk4/2, cfblk6/3(cfblk9)
  cfblk7/1(cfblk2) -> cfblk15/1
  cfblk15/1 -> cfblk8/1(cfblk1)
  cfblk16/1 -> cfblk6/4(cfblk10)
  cfblk8/2(cfblk15) -> cfblk17/1
  cfblk17/1 -> cfblk9/3(cfblk7)
  cfblk18/1 -> cfblk8/3(cfblk13)
  cfblk19/1 -> cfblk11/2(cfblk15)

== system sampleModel1488/cfblk161 ==
  cfblk1 : Inport
  cfblk6 : Inport  Port=2
  cfblk7 : Inport  Port=3
  cfblk8 : Inport  Port=4
  cfblk10 : Delay  SampleTime=1
  cfblk3 : Reshape
  cfblk4 : Subsystem
  cfblk5 : Subsystem
  cfblk2 : Outport
  cfblk9 : Outport  Port=2
  wires:
  cfblk1/1 -> cfblk5/1(cfblk1), cfblk4/4(cfblk15)
  cfblk8/1 -> cfblk4/1(cfblk1)
  cfblk7/1 -> cfblk5/2(cfblk7)
  cfblk6/1 -> cfblk4/2(cfblk13)
  cfblk3/1 -> cfblk9/1
  cfblk5/1(cfblk2) -> cfblk2/1
  cfblk5/2(cfblk9) -> cfblk3/1
  cfblk5/3(cfblk10) -> cfblk4/3(cfblk14)
  cfblk4/1(cfblk2) -> cfblk10/1
  cfblk10/1 -> cfblk5/3(cfblk8)

== system sampleModel1488/cfblk162 ==
  cfblk1 : Inport
  cfblk9 : Inport  Port=2
  cfblk10 : Inport  Port=3
  cfblk11 : Inport  Port=4
  cfblk12 : Delay  SampleTime=1
  cfblk13 : Delay  SampleTime=1
  cfblk3 : ComplexToRealImag
  cfblk4 : Trigonometry
  cfblk5 : Abs  SaturateOnIntegerOverflow=off
  cfblk6 : MinMax  Function=max
  cfblk7 : Subsystem
  cfblk8 : Subsystem
  cfblk2 : Outport
  wires:
  cfblk9/1 -> cfblk7/1(cfblk1)
  cfblk6/1 -> cfblk3/1
  cfblk10/1 -> cfblk5/1
  cfblk1/1 -> cfblk6/1
  cfblk3/1 -> cfblk7/2(cfblk11)
  cfblk11/1 -> cfblk2/1
  cfblk7/1(cfblk2) -> cfblk8/1(cfblk1)
  cfblk5/1 -> cfblk8/2(cfblk6), cfblk7/6(cfblk15)
  cfblk8/1(cfblk2) -> cfblk4/1
  cfblk3/2 -> cfblk7/3(cfblk12)
  cfblk4/1 -> cfblk12/1
  cfblk12/1 -> cfblk7/4(cfblk13)
  cfblk8/2(cfblk7) -> cfblk13/1
  cfblk13/1 -> cfblk7/5(cfblk14)

== system sampleModel1488/cfblk163 ==
  cfblk1 : Inport
  cfblk8 : Inport  Port=2
  cfblk9 : Inport  Port=3
  cfblk10 : Delay  SampleTime=1
  cfblk3 : simulink/Discrete/Tapped Delay  vinit=0.0  samptime=-1  NumDelays=1  DelayOrder=Oldest  includeCurrent=off
  cfblk4 : Sin  TimeSource=Use external signal  SampleTime=0
  cfblk5 : Polyval  Coefs=[ +2.081618890e-019, -1.441693666e-014, +4.719686976e-010, -8.536869453e-006, +1.621573104e-001, -8.087801117e+001 ]
  cfblk6 : Trigonometry
  cfblk7 : Math  Operator=conj
  cfblk2 : Outport
  wires:
  cfblk5/1 -> cfblk6/1
  cfblk1/1 -> cfblk2/1
  cfblk3/1 -> cfblk4/1
  cfblk9/1 -> cfblk7/1
  cfblk8/1 -> cfblk3/1
  cfblk6/1 -> cfblk10/1
  cfblk10/1 -> cfblk5/1

== system sampleModel1488/cfblk164 ==
  cfblk1 : Inport
  cfblk8 : Inport  Port=2
  cfblk10 : Subsystem  TreatAsAtomicUnit=on
  cfblk{11..14} (4 alike) : Delay  SampleTime=1
  cfblk3 : Sin  TimeSource=Use external signal  SampleTime=0
  cfblk4 : Polyval  Coefs=[ +2.081618890e-019, -1.441693666e-014, +4.719686976e-010, -8.536869453e-006, +1.621573104e-001, -8.087801117e+001 ]
  cfblk5 : Subsystem
  cfblk6 : Subsystem
  cfblk7 : If  IfExpression=u1 >= 0  SampleTime=1
  cfblk9 : Subsystem  TreatAsAtomicUnit=on
  cfblk2 : Outport
  wires:
  cfblk10/1(cfblk2) -> cfblk3/1
  cfblk8/1 -> cfblk4/1
  cfblk5/1(cfblk2) -> cfblk7/1
  cfblk9/1(cfblk2) -> cfblk10/1(cfblk1)
  cfblk1/1 -> cfblk5/2(cfblk8), cfblk6/1(cfblk1), cfblk9/4(cfblk14)
  cfblk4/1 -> cfblk9/1(cfblk1)
  cfblk9/2(cfblk15) -> cfblk10/2(cfblk10), cfblk6/2(cfblk15)
  cfblk6/1(cfblk2) -> cfblk2/1
  cfblk7/1 -> cfblk9/Action
  cfblk7/2 -> cfblk10/Action
  cfblk3/1 -> cfblk11/1
  cfblk11/1 -> cfblk5/1(cfblk1)
  cfblk10/2(cfblk12) -> cfblk12/1
  cfblk12/1 -> cfblk9/2(cfblk12)
  cfblk6/2(cfblk16) -> cfblk13/1
  cfblk13/1 -> cfblk10/3(cfblk11)
  cfblk6/3(cfblk17) -> cfblk14/1
  cfblk14/1 -> cfblk9/3(cfblk13)

== system sampleModel1488/cfblk165 ==
  cfblk1 : Inport
  cfblk9 : Inport  Port=2
  cfblk10 : Delay  SampleTime=1
  cfblk11 : Delay  SampleTime=1
  cfblk3 : slpidlib/PID Controller  Controller=PID  Form=Parallel  TimeDomain=Discrete-time  UseExternalTs=off  SampleTime=1  IntegratorMethod=Forward Euler  FilterMethod=Forward Euler  ControllerParametersSource=internal  P=1  I=1  UseKiTs=off  D=0  N=100  UseFilter=on  TunerSelectOption=Transfer Function Based (PID Tuner App)  InitialConditionSource=internal  InitialConditionForIntegrator=0  InitialConditionForFilter=0  DifferentiatorICPrevScaledInput=0  ExternalReset=none  TrackingMode=off  Kt=1  LimitOutput=off  SatLimitsSource=internal  UpperSaturationLimit=inf  LowerSaturationLimit=-inf  LinearizeAsGain=off  AntiWindupMode=none  Kb=1  LimitIntegrator=off  UpperIntegratorSaturationLimit=inf  LowerIntegratorSaturationLimit=-inf  POutMin=[]  POutMax=[]  IOutMin=[]  IOutMax=[]  DOutMin=[]  DOutMax=[]  NOutMin=[]  NOutMax=[]  SumOutMin=[]  SumOutMax=[]  SaturationOutMin=[]  SaturationOutMax=[]  PParamMin=[]  PParamMax=[]  IParamMin=[]  IParamMax=[]  DParamMin=[]  DParamMax=[]  NParamMin=[]  NParamMax=[]  KbParamMin=[]  KbParamMax=[]  KtParamMin=[]  KtParamMax=[]  KbOutMin=[]  KbOutMax=[]  KtOutMin=[]  KtOutMax=[]  IntegratorOutMin=[]  IntegratorOutMax=[]  FilterOutMin=[]  FilterOutMax=[]  SumI1OutMin=[]  SumI1OutMax=[]  SumI2OutMin=[]  SumI2OutMax=[]  SumI3OutMin=[]  SumI3OutMax=[]  SumI4OutMin=[]  SumI4OutMax=[]  SumDOutMin=[]  SumDOutMax=[]  DifferentiatorOutMin=[]  DifferentiatorOutMax=[]  FilterDiffOutCoefMin=[]  FilterDiffOutCoefMax=[]  ReciprocalOutMin=[]  ReciprocalOutMax=[]  SumDenOutMin=[]  SumDenOutMax=[]  SumNumOutMin=[]  SumNumOutMax=[]  DivideOutMin=[]  DivideOutMax=[]  UdiffTsProdOutMin=[]  UdiffTsProdOutMax=[]  NTsProdOutMin=[]  NTsProdOutMax=[]  UintegralTsProdOutMin=[]  UintegralTsProdOutMax=[]  UngainTsProdOutMin=[]  UngainTsProdOutMax=[]  ClampingZeroOutDataTypeStr=Inherit: Inherit via back propagation  ClampingZeroOutMin=[]  ClampingZeroOutMax=[]  FilterDenConstantOutDataTypeStr=Inherit: Inherit via back propagation  FilterDenConstantOutMin=[]  FilterDenConstantOutMax=[]  PCopyOutDataTypeStr=Inherit: Inherit via back propagation  PCopyOutMin=[]  PCopyOutMax=[]  NCopyOutDataTypeStr=Inherit: Inherit via back propagation  NCopyOutMin=[]  NCopyOutMax=[]  IntegratorContinuousStateAttributes=''  IntegratorStateMustResolveToSignalObject=off  IntegratorRTWStateStorageClass=Auto  FilterContinuousStateAttributes=''  FilterStateMustResolveToSignalObject=off  FilterRTWStateStorageClass=Auto  ParallelPVariant=InternalParameters  IdealPVariant=Disabled  IVariant=InternalParameters  DVariant=InternalParameters  IntegratorVariant=Discrete  SatVariant=Disabled  AWVariant=Passthrough  PCopyVariant=Disabled  TRVariant=Disabled  FdbkBlocksVariant=Forward  IdealPFdbkVariant=Disabled  SatFdbkVariant=Disabled  DerivativeFilterVariant=ForwardEulerFilter  NVariant=InternalParameters  NCopyVariant=Disabled  FilterICVariant=InternalICsFilter  IntegratorICVariant=InternalICs  ExternalResetVariant=Disabled  TRSumVariant=Passthrough  SumFdbkVariant=Disabled  SumVariant=Sum_PID  TsampFilterVariant=InternalTs  TsampNgainVariant=Passthrough  TsampIntegralVariant=Disabled_SignalSpec  ExternalSaturationOutDataTypeStr=Inherit: Same as second input
      settings: LibrarySourceBlock=simulink/Discrete/Discrete PID Controller
  cfblk4 : simulink/Discrete/Tapped Delay  vinit=0.0  samptime=-1  NumDelays=1  DelayOrder=Oldest  includeCurrent=off
  cfblk5 : Constant  Value=[382221393.018636]  SampleTime=1
  cfblk6 : Subsystem
  cfblk7 : Subsystem
  cfblk8 : Subsystem
  cfblk2 : Outport
  wires:
  cfblk6/1(cfblk2) -> cfblk4/1
  cfblk3/1 -> cfblk7/1(cfblk1)
  cfblk5/1 -> cfblk3/1, cfblk8/4(cfblk13), cfblk6/4(cfblk13)
  cfblk8/1(cfblk2) -> cfblk2/1
  cfblk6/2(cfblk15) -> cfblk7/2(cfblk13)
  cfblk4/1 -> cfblk8/1(cfblk1), cfblk8/5(cfblk14), cfblk8/6(cfblk15)
  cfblk7/1(cfblk2) -> cfblk8/2(cfblk11)
  cfblk9/1 -> cfblk8/3(cfblk12), cfblk6/5(cfblk14)
  cfblk1/1 -> cfblk6/1(cfblk1)
  cfblk8/2(cfblk16) -> cfblk10/1
  cfblk10/1 -> cfblk6/2(cfblk11)
  cfblk7/2(cfblk14) -> cfblk11/1
  cfblk11/1 -> cfblk6/3(cfblk12)

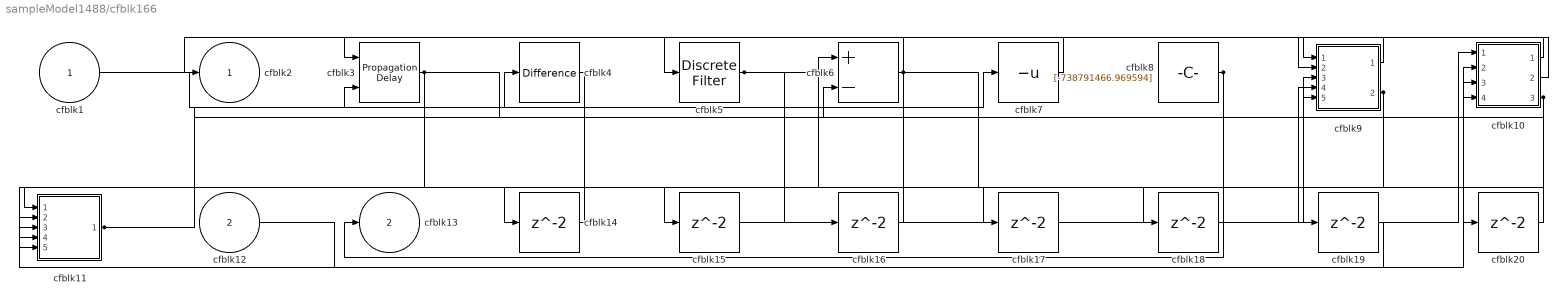
== system sampleModel1488/cfblk166 ==
  cfblk1 : Inport
  cfblk12 : Inport  Port=2
  cfblk10 : Subsystem
  cfblk11 : Subsystem
  cfblk{14..20} (7 alike) : Delay  SampleTime=1
  cfblk3 : PropagationDelay  SampleTime=1
  cfblk4 : simulink/Discrete/Difference  ICPrevInput=0.0  OutMin=[]  OutMax=[]  OutDataTypeStr=Inherit: Inherit via back propagation  OutDataType=fixdt(1, 16)  OutScaling=2^-10  DoSatur=off
  cfblk5 : DiscreteFilter  SampleTime=1
  cfblk6 : Sum  Inputs=+-
  cfblk7 : UnaryMinus
  cfblk8 : Constant  Value=[-738791466.969594]  SampleTime=1
  cfblk9 : Subsystem
  cfblk2 : Outport
  cfblk13 : Outport  Port=2
  wires:
  cfblk7/1 -> cfblk3/1
  cfblk1/1 -> cfblk7/1
  cfblk11/1(cfblk2) -> cfblk4/1, cfblk10/3(cfblk14)
  cfblk10/1(cfblk2) -> cfblk9/1(cfblk1)
  cfblk6/1 -> cfblk5/1, cfblk15/1, cfblk18/1
  cfblk3/1 -> cfblk11/1(cfblk1), cfblk10/4(cfblk15), cfblk11/5(cfblk13)
  cfblk8/1 -> cfblk13/1, cfblk11/2(cfblk10)
  cfblk5/1 -> cfblk16/1, cfblk17/1
  cfblk12/1 -> cfblk10/2(cfblk13)
  cfblk10/2(cfblk16) -> cfblk9/2(cfblk11)
  cfblk10/3(cfblk17) -> cfblk9/3(cfblk12), cfblk20/1
  cfblk9/1(cfblk2) -> cfblk2/1
  cfblk9/2(cfblk15) -> cfblk6/2, cfblk19/1
  cfblk4/1 -> cfblk14/1
  cfblk14/1 -> cfblk3/2
  cfblk15/1 -> cfblk10/1(cfblk1)
  cfblk16/1 -> cfblk6/1
  cfblk17/1 -> cfblk9/4(cfblk13)
  cfblk18/1 -> cfblk9/5(cfblk14)
  cfblk19/1 -> cfblk11/4(cfblk12)
  cfblk20/1 -> cfblk11/3(cfblk11)

== system sampleModel1488/cfblk167 ==
  cfblk1 : Inport
  cfblk13 : Inport  Port=2
  cfblk14 : Inport  Port=3
  cfblk15 : Inport  Port=4
  cfblk10 : Subsystem
  cfblk11 : Subsystem
  cfblk12 : Subsystem
  cfblk18 : simulink_need_slupdate/First-Order Hold  DisableCoverage=on  Ts=1
  cfblk19 : simulink_need_slupdate/First-Order Hold  DisableCoverage=on  Ts=1
  cfblk3 : DiscreteZeroPole  Poles=[0 0.5]  Gain=1
  cfblk4 : simulink/Discrete/Transfer Fcn First Order  PoleZ=0.95  ICPrevOutput=0.0  DoSatur=off
  cfblk5 : Sum  Inputs=|++
  cfblk6 : Constant  Value=[861979675.632754]  SampleTime=1
  cfblk7 : Constant  Value=[218491970.947063]  SampleTime=1
  cfblk8 : Constant  Value=[-515912650.524280]  SampleTime=1
  cfblk9 : Constant  Value=[-437131248.001230]  SampleTime=1
  cfblk2 : Outport
  cfblk16 : Outport  Port=2
  cfblk17 : Outport  Port=3
  wires:
  cfblk4/1 -> cfblk11/1(cfblk1)
  cfblk13/1 -> cfblk3/1
  cfblk7/1 -> cfblk2/1
  cfblk12/1(cfblk2) -> cfblk11/2(cfblk8)
  cfblk6/1 -> cfblk16/1
  cfblk8/1 -> cfblk17/1
  cfblk12/2(cfblk12) -> cfblk4/1
  cfblk3/1 -> cfblk10/1(cfblk1)
  cfblk1/1 -> cfblk12/1(cfblk1)
  cfblk5/1 -> cfblk10/2(cfblk8)
  cfblk15/1 -> cfblk18/1
  cfblk18/1 -> cfblk5/1
  cfblk9/1 -> cfblk19/1
  cfblk19/1 -> cfblk5/2

== system sampleModel1488/cfblk168 ==
  cfblk1 : Inport
  cfblk9 : Inport  Port=2
  cfblk12 : Delay  SampleTime=1
  cfblk3 : simulink/Math Operations/Slider Gain  gain=1  low=0  high=2
  cfblk4 : simulink/Math Operations/MinMax Running Resettable  Function=min  vinit=0.0
  cfblk5 : Sum  Inputs=|++
  cfblk6 : Sqrt  Operator=rSqrt  AlgorithmType=Newton-Raphson
  cfblk7 : Constant  Value=[-897312050.701647]  SampleTime=1
  cfblk8 : Subsystem
  cfblk2 : Outport
  cfblk10 : Outport  Port=2
  cfblk11 : Outport  Port=3
  wires:
  cfblk4/1 -> cfblk6/1
  cfblk7/1 -> cfblk3/1, cfblk8/5(cfblk11)
  cfblk3/1 -> cfblk11/1, cfblk8/6(cfblk12)
  cfblk5/1 -> cfblk10/1
  cfblk1/1 -> cfblk8/1(cfblk1), cfblk8/3(cfblk9), cfblk8/4(cfblk10)
  cfblk9/1 -> cfblk8/2(cfblk8)
  cfblk8/1(cfblk2) -> cfblk5/1
  cfblk8/2(cfblk13) -> cfblk2/1
  cfblk8/3(cfblk14) -> cfblk4/2
  cfblk8/4(cfblk15) -> cfblk5/2
  cfblk6/1 -> cfblk12/1
  cfblk12/1 -> cfblk4/1

== system sampleModel1488/cfblk169 ==
  cfblk1 : Inport
  cfblk11 : Delay  SampleTime=1
  cfblk3 : DiscreteTransferFcn  SampleTime=1
  cfblk4 : simulink/Discrete/Transfer Fcn First Order  PoleZ=0.95  ICPrevOutput=0.0  DoSatur=off
  cfblk5 : Sum  Inputs=--
  cfblk6 : Subsystem
  cfblk7 : Subsystem
  cfblk8 : Subsystem
  cfblk2 : Outport
  cfblk9 : Outport  Port=2
  cfblk10 : Outport  Port=3
  wires:
  cfblk6/1(cfblk2) -> cfblk10/1
  cfblk4/1 -> cfblk8/1(cfblk1)
  cfblk5/1 -> cfblk7/1(cfblk1)
  cfblk8/1(cfblk2) -> cfblk6/1(cfblk1)
  cfblk3/1 -> cfblk9/1
  cfblk6/2(cfblk14) -> cfblk5/1
  cfblk8/2(cfblk7) -> cfblk5/2, cfblk3/1
  cfblk1/1 -> cfblk2/1
  cfblk7/1(cfblk2) -> cfblk11/1
  cfblk11/1 -> cfblk4/1

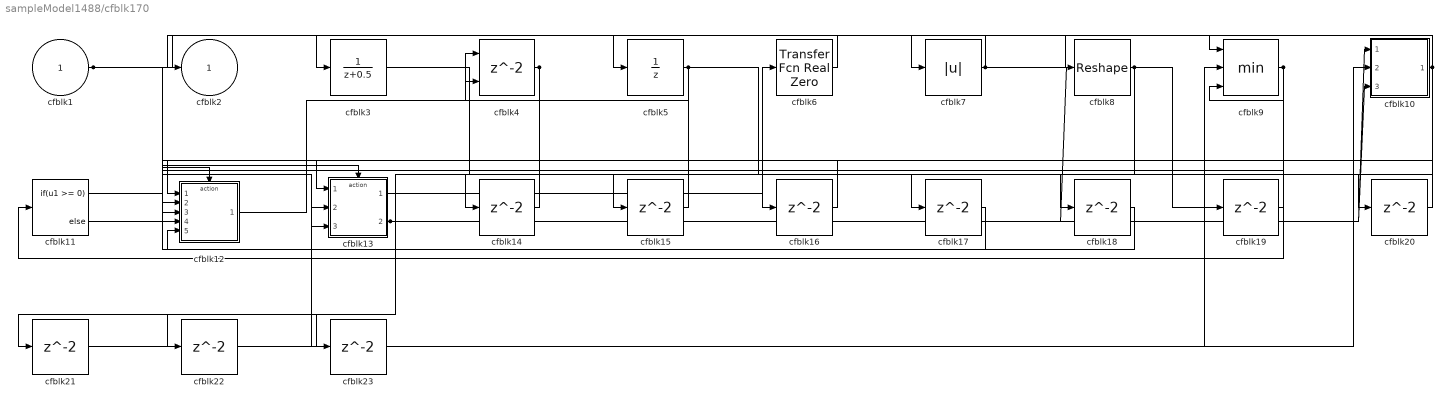
== system sampleModel1488/cfblk170 ==
  cfblk1 : Inport
  cfblk10 : Subsystem
  cfblk11 : If  IfExpression=u1 >= 0  SampleTime=1
  cfblk12 : Subsystem  TreatAsAtomicUnit=on
  cfblk13 : Subsystem  TreatAsAtomicUnit=on
  cfblk{14..23} (10 alike) : Delay  SampleTime=1
  cfblk3 : DiscreteTransferFcn  SampleTime=1
  cfblk4 : Delay  ShowEnablePort=on  SampleTime=1
      settings: InputPortMap=u0,e6
  cfblk5 : UnitDelay  HasFrameUpgradeWarning=on
  cfblk6 : simulink/Discrete/Transfer Fcn Real Zero  ZeroZ=0.75  ICPrevInput=0.0  DoSatur=off
  cfblk7 : Abs  SaturateOnIntegerOverflow=off
  cfblk8 : Reshape
  cfblk9 : MinMax  Inputs=3
  cfblk2 : Outport
  wires:
  cfblk10/1(cfblk2) -> cfblk5/1, cfblk22/1
  cfblk4/1 -> cfblk14/1, cfblk23/1
  cfblk5/1 -> cfblk20/1, cfblk21/1
  cfblk9/1 -> cfblk11/1, cfblk12/4(cfblk14)
  cfblk6/1 -> cfblk3/1
  cfblk13/1(cfblk2) -> cfblk6/1
  cfblk12/1(cfblk2) -> cfblk4/1
  cfblk1/1 -> cfblk7/1, cfblk13/3(cfblk8)
  cfblk8/1 -> cfblk16/1, cfblk17/1, cfblk18/1, cfblk19/1
  cfblk7/1 -> cfblk9/1, cfblk2/1
  cfblk13/2(cfblk9) -> cfblk8/1, cfblk10/1(cfblk1), cfblk10/3(cfblk11)
  cfblk11/1 -> cfblk12/Action
  cfblk11/2 -> cfblk13/Action
  cfblk14/1 -> cfblk13/1(cfblk1)
  cfblk3/1 -> cfblk15/1
  cfblk15/1 -> cfblk4/2
  cfblk16/1 -> cfblk12/2(cfblk12)
  cfblk17/1 -> cfblk12/3(cfblk13)
  cfblk18/1 -> cfblk12/5(cfblk15)
  cfblk19/1 -> cfblk9/3
  cfblk20/1 -> cfblk12/1(cfblk1)
  cfblk21/1 -> cfblk10/2(cfblk10)
  cfblk22/1 -> cfblk13/2(cfblk7)
  cfblk23/1 -> cfblk9/2

== system sampleModel1488/cfblk171 ==
  cfblk1 : Inport
  cfblk{9..12} (4 alike) : Delay  SampleTime=1
  cfblk3 : DiscreteIntegrator  ICPrevOutput=DiscIntNeverNeededParam  ICPrevScaledInput=DiscIntNeverNeededParam
  cfblk4 : Product  Inputs=*
  cfblk5 : Abs  SaturateOnIntegerOverflow=off
  cfblk6 : Subsystem
  cfblk7 : Subsystem
  cfblk2 : Outport
  cfblk8 : Outport  Port=2
  wires:
  cfblk6/1(cfblk2) -> cfblk4/1
  cfblk6/2(cfblk14) -> cfblk5/1
  cfblk3/1 -> cfblk8/1, cfblk10/1, cfblk11/1
  cfblk7/2(cfblk9) -> cfblk3/1
  cfblk4/1 -> cfblk2/1, cfblk7/2(cfblk7), cfblk7/3(cfblk8)
  cfblk1/1 -> cfblk6/2(cfblk11)
  cfblk7/1(cfblk2) -> cfblk9/1
  cfblk9/1 -> cfblk6/1(cfblk1)
  cfblk10/1 -> cfblk7/1(cfblk1)
  cfblk11/1 -> cfblk6/4(cfblk13)
  cfblk5/1 -> cfblk12/1
  cfblk12/1 -> cfblk6/3(cfblk12)

== system sampleModel1488/cfblk172 ==
  cfblk1 : Inport
  cfblk13 : Inport  Port=2
  cfblk14 : Inport  Port=3
  cfblk10 : Subsystem
  cfblk11 : Subsystem
  cfblk12 : Subsystem
  cfblk15 : Delay  SampleTime=1
  cfblk3 : slpidlib/PID Controller  Controller=PID  Form=Parallel  TimeDomain=Discrete-time  UseExternalTs=off  SampleTime=1  IntegratorMethod=Forward Euler  FilterMethod=Forward Euler  ControllerParametersSource=internal  P=1  I=1  UseKiTs=off  D=0  N=100  UseFilter=on  TunerSelectOption=Transfer Function Based (PID Tuner App)  InitialConditionSource=internal  InitialConditionForIntegrator=0  InitialConditionForFilter=0  DifferentiatorICPrevScaledInput=0  ExternalReset=none  TrackingMode=off  Kt=1  LimitOutput=off  SatLimitsSource=internal  UpperSaturationLimit=inf  LowerSaturationLimit=-inf  LinearizeAsGain=off  AntiWindupMode=none  Kb=1  LimitIntegrator=off  UpperIntegratorSaturationLimit=inf  LowerIntegratorSaturationLimit=-inf  POutMin=[]  POutMax=[]  IOutMin=[]  IOutMax=[]  DOutMin=[]  DOutMax=[]  NOutMin=[]  NOutMax=[]  SumOutMin=[]  SumOutMax=[]  SaturationOutMin=[]  SaturationOutMax=[]  PParamMin=[]  PParamMax=[]  IParamMin=[]  IParamMax=[]  DParamMin=[]  DParamMax=[]  NParamMin=[]  NParamMax=[]  KbParamMin=[]  KbParamMax=[]  KtParamMin=[]  KtParamMax=[]  KbOutMin=[]  KbOutMax=[]  KtOutMin=[]  KtOutMax=[]  IntegratorOutMin=[]  IntegratorOutMax=[]  FilterOutMin=[]  FilterOutMax=[]  SumI1OutMin=[]  SumI1OutMax=[]  SumI2OutMin=[]  SumI2OutMax=[]  SumI3OutMin=[]  SumI3OutMax=[]  SumI4OutMin=[]  SumI4OutMax=[]  SumDOutMin=[]  SumDOutMax=[]  DifferentiatorOutMin=[]  DifferentiatorOutMax=[]  FilterDiffOutCoefMin=[]  FilterDiffOutCoefMax=[]  ReciprocalOutMin=[]  ReciprocalOutMax=[]  SumDenOutMin=[]  SumDenOutMax=[]  SumNumOutMin=[]  SumNumOutMax=[]  DivideOutMin=[]  DivideOutMax=[]  UdiffTsProdOutMin=[]  UdiffTsProdOutMax=[]  NTsProdOutMin=[]  NTsProdOutMax=[]  UintegralTsProdOutMin=[]  UintegralTsProdOutMax=[]  UngainTsProdOutMin=[]  UngainTsProdOutMax=[]  ClampingZeroOutDataTypeStr=Inherit: Inherit via back propagation  ClampingZeroOutMin=[]  ClampingZeroOutMax=[]  FilterDenConstantOutDataTypeStr=Inherit: Inherit via back propagation  FilterDenConstantOutMin=[]  FilterDenConstantOutMax=[]  PCopyOutDataTypeStr=Inherit: Inherit via back propagation  PCopyOutMin=[]  PCopyOutMax=[]  NCopyOutDataTypeStr=Inherit: Inherit via back propagation  NCopyOutMin=[]  NCopyOutMax=[]  IntegratorContinuousStateAttributes=''  IntegratorStateMustResolveToSignalObject=off  IntegratorRTWStateStorageClass=Auto  FilterContinuousStateAttributes=''  FilterStateMustResolveToSignalObject=off  FilterRTWStateStorageClass=Auto  ParallelPVariant=InternalParameters  IdealPVariant=Disabled  IVariant=InternalParameters  DVariant=InternalParameters  IntegratorVariant=Discrete  SatVariant=Disabled  AWVariant=Passthrough  PCopyVariant=Disabled  TRVariant=Disabled  FdbkBlocksVariant=Forward  IdealPFdbkVariant=Disabled  SatFdbkVariant=Disabled  DerivativeFilterVariant=ForwardEulerFilter  NVariant=InternalParameters  NCopyVariant=Disabled  FilterICVariant=InternalICsFilter  IntegratorICVariant=InternalICs  ExternalResetVariant=Disabled  TRSumVariant=Passthrough  SumFdbkVariant=Disabled  SumVariant=Sum_PID  TsampFilterVariant=InternalTs  TsampNgainVariant=Passthrough  TsampIntegralVariant=Disabled_SignalSpec  ExternalSaturationOutDataTypeStr=Inherit: Same as second input
      settings: LibrarySourceBlock=simulink/Discrete/Discrete PID Controller
  cfblk4 : PropagationDelay  SampleTime=1
  cfblk5 : simulink/Discrete/Transfer Fcn First Order  PoleZ=0.95  ICPrevOutput=0.0  DoSatur=off
  cfblk6 : simulink/Discrete/Tapped Delay  vinit=0.0  samptime=-1  NumDelays=1  DelayOrder=Oldest  includeCurrent=off
  cfblk7 : Sum  Inputs=+-
  cfblk8 : Reshape
  cfblk9 : Constant  Value=[-718419582.295529]  SampleTime=1
  cfblk2 : Outport
  wires:
  cfblk3/1 -> cfblk5/1, cfblk11/2(cfblk7)
  cfblk1/1 -> cfblk8/1
  cfblk8/1 -> cfblk7/2, cfblk12/2(cfblk14), cfblk12/3(cfblk15), cfblk12/4(cfblk16)
  cfblk5/1 -> cfblk10/1(cfblk1)
  cfblk10/1(cfblk2) -> cfblk4/1
  cfblk13/1 -> cfblk10/2(cfblk8)
  cfblk4/1 -> cfblk6/1
  cfblk9/1 -> cfblk10/3(cfblk9)
  cfblk7/1 -> cfblk11/1(cfblk1), cfblk11/3(cfblk8)
  cfblk11/1(cfblk2) -> cfblk12/1(cfblk1)
  cfblk12/1(cfblk2) -> cfblk4/2
  cfblk14/1 -> cfblk3/1
  cfblk12/2(cfblk17) -> cfblk2/1
  cfblk6/1 -> cfblk15/1
  cfblk15/1 -> cfblk7/1
